simulink model "mfcMultiUnitDeltaVar"  (R2015a)
settings: Solver=ode15s  StartTime=0.0  StopTime=4000  RelTol=1e-6  AbsTol=1e-9
InitFcn:
  | delta = 20;
  | kmu = 20000;
  | 
  | beta = 0;
  | %beta = -10;
  | gamma = 0;
  | gamma = 5;
  | 
  | dummy = 0;
  | 
  | Rinit = 200;
settings Model: Creator=ironi  LastModifiedBy=ironi
settings HardwareCC: ProdBitPerLong=64  ProdBitPerPointer=64  ProdWordSize=64  ProdHWDeviceType=Generic->64-bit Embedded Processor (LP64)

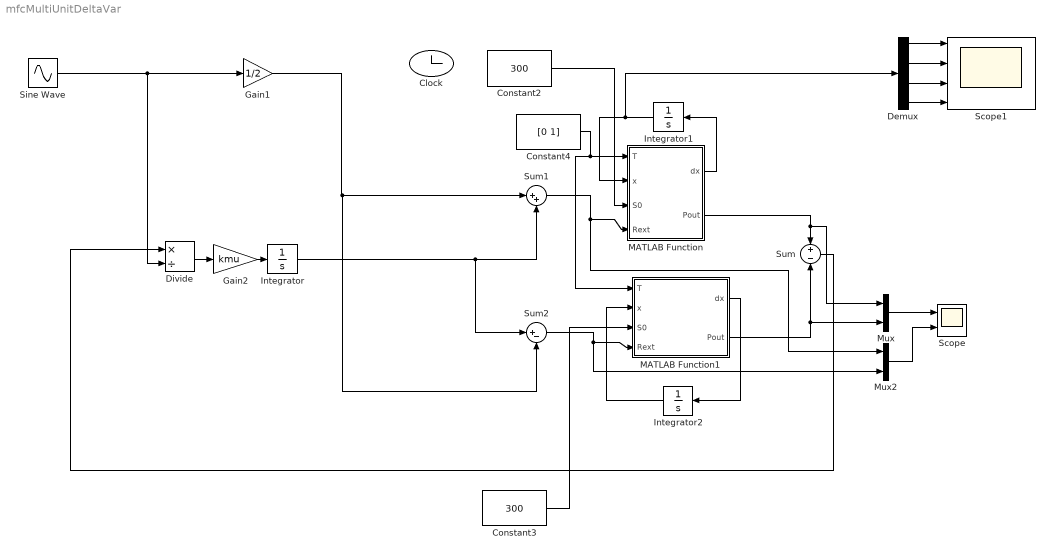
== system mfcMultiUnitDeltaVar ==
  Clock : Clock
  Constant2 : Constant  Value=300
  Constant3 : Constant  Value=300
  Constant4 : Constant  Value=[0 1]
  Demux : Demux
  Divide : Product  Inputs=*/
  Gain1 : Gain  Gain=1/2
  Gain2 : Gain  Gain=kmu
  Integrator : Integrator  InitialCondition=Rinit
  Integrator1 : Integrator  InitialCondition="[20.8395  498.2432    2.0000    0.0412]"
  Integrator2 : Integrator  InitialCondition="[20.8395  498.2432    2.0000    0.0412]"
  MATLAB Function : MATLAB Function  TreatAsAtomicUnit=on
  MATLAB Function1 : MATLAB Function  TreatAsAtomicUnit=on
  Mux : Mux  Inputs=2
  Mux2 : Mux  Inputs=2
  Scope : Scope  NumInputPorts=2
      settings: YMin=0.00172~147  YMax=0.001734~168
  Scope1 : Scope  NumInputPorts=4
      settings: YMin=-5~-5~-5~-5  YMax=5~5~5~5
  Sine Wave : Sin  Amplitude=20  Bias=20  Frequency=1/999  SampleTime=0
  Sum : Sum  Inputs=+|-
  Sum1 : Sum  Inputs=|++
  Sum2 : Sum  Inputs=|+-
  wires:
  Sum/1 -> Divide/1
  Divide/1 -> Gain2/1
  Sum1/1 -> MATLAB Function/4(Rext), Mux2/1
  Mux/1 -> Scope/1
  Gain1/1 -> Sum2/2, Sum1/1
  Sum2/1 -> MATLAB Function1/4(Rext), Mux2/2
  MATLAB Function/1(dx) -> Integrator1/1
  Mux2/1 -> Scope/2
  MATLAB Function1/2(Pout) -> Mux/2, Sum/2
  MATLAB Function/2(Pout) -> Mux/1, Sum/1
  Integrator1/1 -> Demux/1, MATLAB Function/2(x)
  MATLAB Function1/1(dx) -> Integrator2/1
  Integrator2/1 -> MATLAB Function1/2(x)
  Constant4/1 -> MATLAB Function1/1(T), MATLAB Function/1(T)
  Constant2/1 -> MATLAB Function/3(S0)
  Constant3/1 -> MATLAB Function1/3(S0)
  Demux/2 -> Scope1/2
  Demux/1 -> Scope1/1
  Demux/3 -> Scope1/3
  Demux/4 -> Scope1/4
  Integrator/1 -> Sum2/1, Sum1/2
  Sine Wave/1 -> Divide/2, Gain1/1
  Gain2/1 -> Integrator/1

== matlab function mfcMultiUnitDeltaVar/MATLAB Function1 ==
  data: T input; dx output; x input; dummy parameter; S0 input; Rext input; Pout output
function [dx, Pout]= mfcModel(T, x, dummy, S0, Rext)
F = 96485;
R = 8.314472;
T = 298.15;
Y = 22.753;
Ych4 = .3;
qmax_a = 8.48;
qmax_m = 8.2;
umax_a = 1.9753;
umax_m = .1;
Ks_a = 20;
Ks_m = 80;
m = 2;
gamma = 663400;
Mtotal = .05;
Km = .2*Mtotal;
Kd_a = .02*umax_a;
Kd_m = .02*umax_m;
Xmax_a = 512.5;
Xmax_m = 537.5;
Kx = .04;
Rmin = 25;
Rmax = 2000 + Rmin;
Emin = .01;
Emax = 0.25 + 0.4144+ Emin;
Kr = .024;

i0ref=0.4*4;

e = 0.0001*Mtotal;

V = 0.05;
Fin = 0.1527;

D = Fin/V;

S   = x(1);
xa  = x(2);
xm  = x(3);
Mox = x(4);

%% Équations dynamiques
  
Mred = Mtotal - Mox;

Rint = Rmin + (Rmax - Rmin) * exp(-Kr*xa);                          % (22)
Eocv = Emin + (Emax - Emin) * exp(-1/(Kr*xa));                      % (23)

alpha_a = 1/2*(1 + tanh(Kx*(xa + xm - Xmax_a)));                    % (9)
alpha_m = 1/2*(1 + tanh(Kx*(xa + xm - Xmax_m)));                    % (9)

qa = qmax_a * S / (Ks_a + S) * Mox / (Km + Mox);                    % (15)
qm = qmax_m * S / (Ks_m + S);                                       % (16)

ua = umax_a * S / (Ks_a + S) * Mox / (Km + Mox);                    % (13)
um = umax_m * S / (Ks_m + S);                                       % (14)

n_conc = R*T/F/m * log(Mtotal/Mred);                                % (18)

Imfc = (Eocv - n_conc) / (Rext + Rint) * Mred / (e + Mred);         % (21)

Sp = -qa*xa - qm*xm + D*(S0 - S);                                   % (6)
Xap = ua*xa - Kd_a*xa - alpha_a*D*xa;                               % (7)
Xmp = um*xm - Kd_m*xm - alpha_m*D*xm;                               % (8)

Moxp = -Y*qa + gamma*Imfc / (m*F*V*xa) * 86400;                     % (12)

if xa < 1 && Xap < 0
  Xap = 0;
end

if xm < 0.99 && Xmp < 0
  Xmp = 0;
end

Pout = Rext*Imfc^2;

dx = [Sp; Xap; Xmp; Moxp];

== matlab function mfcMultiUnitDeltaVar/MATLAB Function ==
  data: T input; dx output; x input; dummy parameter; S0 input; Rext input; Pout output
function [dx, Pout]= mfcModel(T, x, dummy, S0, Rext)
F = 96485;
R = 8.314472;
T = 298.15;
Y = 22.753;
Ych4 = .3;
qmax_a = 8.48;
qmax_m = 8.2;
umax_a = 1.9753;
umax_m = .1;
Ks_a = 20;
Ks_m = 80;
m = 2;
gamma = 663400;
Mtotal = .05;
Km = .2*Mtotal;
Kd_a = .02*umax_a;
Kd_m = .02*umax_m;
Xmax_a = 512.5;
Xmax_m = 537.5;
Kx = .04;
Rmin = 25;
Rmax = 2000 + Rmin;
Emin = .01;
Emax = 0.25 + 0.4144+ Emin;
Kr = .024;

i0ref=0.4*4;

e = 0.0001*Mtotal;

V = 0.05;
Fin = 0.1527;

D = Fin/V;

S   = x(1);
xa  = x(2);
xm  = x(3);
Mox = x(4);

%% Équations dynamiques
  
Mred = Mtotal - Mox;

Rint = Rmin + (Rmax - Rmin) * exp(-Kr*xa);                          % (22)
Eocv = Emin + (Emax - Emin) * exp(-1/(Kr*xa));                      % (23)

alpha_a = 1/2*(1 + tanh(Kx*(xa + xm - Xmax_a)));                    % (9)
alpha_m = 1/2*(1 + tanh(Kx*(xa + xm - Xmax_m)));                    % (9)

qa = qmax_a * S / (Ks_a + S) * Mox / (Km + Mox);                    % (15)
qm = qmax_m * S / (Ks_m + S);                                       % (16)

ua = umax_a * S / (Ks_a + S) * Mox / (Km + Mox);                    % (13)
um = umax_m * S / (Ks_m + S);                                       % (14)

n_conc = R*T/F/m * log(Mtotal/Mred);                                % (18)

Imfc = (Eocv - n_conc) / (Rext + Rint) * Mred / (e + Mred);         % (21)

Sp = -qa*xa - qm*xm + D*(S0 - S);                                   % (6)
Xap = ua*xa - Kd_a*xa - alpha_a*D*xa;                               % (7)
Xmp = um*xm - Kd_m*xm - alpha_m*D*xm;                               % (8)

Moxp = -Y*qa + gamma*Imfc / (m*F*V*xa) * 86400;                     % (12)

if xa < 1 && Xap < 0
  Xap = 0;
end

if xm < 0.99 && Xmp < 0
  Xmp = 0;
end

Pout = Rext*Imfc^2;

dx = [Sp; Xap; Xmp; Moxp];
